simulink model "BG"  (R2014a)
settings: Solver=ode3  StartTime=0.0  StopTime=1  FixedStep=dt  MaxStep=dt  RelTol=1e-3
values from neighbouring files (symbols this model uses):
  a1 = .4    (= 0.4)    [parameters.m]
  a2 = .35    (= 0.35)    [parameters.m]
  a3 = .25    (= 0.25)    [parameters.m]
  aTc = 0.05    [parameters.m]
  dt = 1e-3    (= 0.001)    [parameters.m]
  g = 1    [parameters.m]
  K = 1    [parameters.m]
  mTc = 0.01    [parameters.m]
  OP1_0 = [ax1_0 ay1_0 0]    [parameters.m]
  OP2_0 = OP1_0 + P1P2_0    [parameters.m]
  OP3_0 = OP2_0 + P2P3_0    [parameters.m]
  OT = [xf yf 0]    [animation.m]    (also in parameters.m = [0.5 0.5 0])
  OT_cercle = [0.6 0.55 0]    [parameters.m]
  p1 = w2 + w3    (= 3)    [parameters.m]
  P1P2_0 = [ax2_0 ay2_0 0]    [parameters.m]
  p2 = w1 + w3    (= 4)    [parameters.m]
  P2P3_0 = [ax3_0 ay3_0 0]    [parameters.m]
  p3 = w2 + w1    (= 5)    [parameters.m]
  tau = 0.001    [parameters.m]
  theta1_0 = zero_vector    [parameters.m]
  theta2_0 = zero_vector    [parameters.m]
  theta3_0 = zero_vector    [parameters.m]
  Vmax = 30    [parameters.m]
  w1 = 3    [parameters.m]
  w2 = 2    [parameters.m]
  w3 = 1    [parameters.m]
  zero_vector = [0 0 0]    [parameters.m]
libraries: vrlib x9, simulink x1
(part 1 of 4)
settings Model: Creator=Armin  LastModifiedBy=Armin

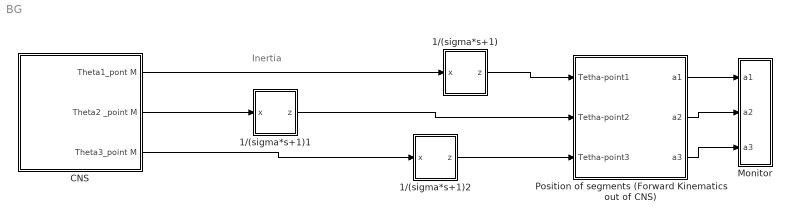
== system BG ==
  note: Inertia
  1/(sigma*s+1) : Subsystem  TreatAsAtomicUnit=on
  1/(sigma*s+1)1 : Subsystem  TreatAsAtomicUnit=on
  1/(sigma*s+1)2 : Subsystem  TreatAsAtomicUnit=on
  CNS : Subsystem
  Monitor : Subsystem
  Position of segments (Forward Kinematics out of CNS) : Subsystem
  wires:
  Position of segments (Forward Kinematics out of CNS)/1(a1) -> Monitor/1(a1)
  Position of segments (Forward Kinematics out of CNS)/2(a2) -> Monitor/2(a2)
  Position of segments (Forward Kinematics out of CNS)/3(a3) -> Monitor/3(a3)
  CNS/1(Theta1_pont M) -> 1/(sigma*s+1)/1(x)
  CNS/2(Theta2 _point M) -> 1/(sigma*s+1)1/1(x)
  CNS/3("Theta3_point M ") -> 1/(sigma*s+1)2/1(x)
  1/(sigma*s+1)/1(z) -> Position of segments (Forward Kinematics out of CNS)/1(Tetha-point1)
  1/(sigma*s+1)2/1(z) -> Position of segments (Forward Kinematics out of CNS)/3(Tetha-point3)
  1/(sigma*s+1)1/1(z) -> Position of segments (Forward Kinematics out of CNS)/2(Tetha-point2)

== system BG/1//(sigma*s+1) ==
  x : Inport
  Add : Sum  Inputs=+-
  Add1 : Sum
  Delay : Delay  DelayLength=1  InitialCondition=zero_vector
  Gain : Gain  Gain=dt
  Gain1 : Gain  Gain=0.9999999
  Gain2 : Gain  Gain=1/0.01
  z : Outport
  wires:
  Add/1 -> Gain/1
  Gain1/1 -> Add1/2, Add/2
  Delay/1 -> Gain1/1
  Gain/1 -> Gain2/1
  x/1 -> Add/1
  Add1/1 -> z/1, Delay/1
  Gain2/1 -> Add1/1

== system BG/1//(sigma*s+1)1 ==
  x : Inport
  Add : Sum  Inputs=+-
  Add1 : Sum
  Delay : Delay  DelayLength=1  InitialCondition=zero_vector
  Gain : Gain  Gain=dt
  Gain1 : Gain  Gain=0.9999999
  Gain2 : Gain  Gain=1/0.01
  z : Outport
  wires:
  Add/1 -> Gain/1
  Gain1/1 -> Add1/2, Add/2
  Delay/1 -> Gain1/1
  Gain/1 -> Gain2/1
  x/1 -> Add/1
  Add1/1 -> z/1, Delay/1
  Gain2/1 -> Add1/1

== system BG/1//(sigma*s+1)2 ==
  x : Inport
  Add : Sum  Inputs=+-
  Add1 : Sum
  Delay : Delay  DelayLength=1  InitialCondition=zero_vector
  Gain : Gain  Gain=dt
  Gain1 : Gain  Gain=0.9999999
  Gain2 : Gain  Gain=1/0.01
  z : Outport
  wires:
  Add/1 -> Gain/1
  Gain1/1 -> Add1/2, Add/2
  Delay/1 -> Gain1/1
  Gain/1 -> Gain2/1
  x/1 -> Add/1
  Add1/1 -> z/1, Delay/1
  Gain2/1 -> Add1/1

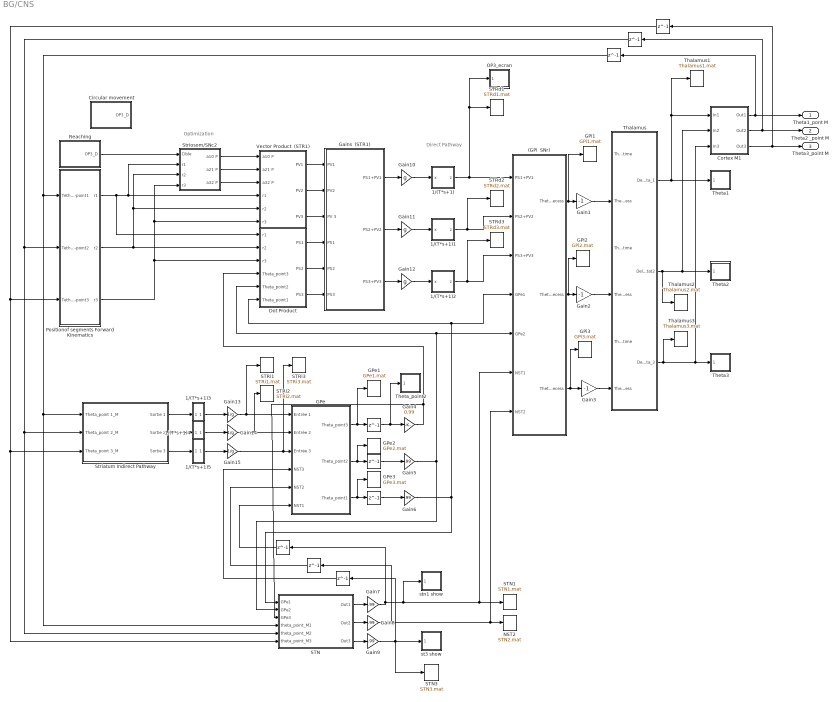
== system BG/CNS ==
  note: Direct Pathway
  note: Optimization
  " (GPi  SNr)" : Subsystem
  " Striosom/SNc2" : Subsystem
  "                                               \t\t\t\t\t\t\t" : Delay  DelayLength=1  InitialCondition=zero_vector
  "                                                                                                                                           " : Delay  DelayLength=1  InitialCondition=zero_vector
  "                                                                                                                                              \t                                                              " : Delay  DelayLength=1  InitialCondition=zero_vector
  "                                                                                                                                              \t                                                               " : Delay  DelayLength=1  InitialCondition=zero_vector
  "                                                                                                                                              \t                                                                " : Delay  DelayLength=1  InitialCondition=zero_vector
  "                                                                                                                                              \t                                                                                " : Delay  DelayLength=1  InitialCondition=zero_vector
  "                                                                                                                                              \t                                                                                    " : Delay  DelayLength=1  InitialCondition=zero_vector
  "                                                                                                                                              \t                                                                                           " : Delay  DelayLength=1  InitialCondition=zero_vector
  "                                                                                                                                                    " : Delay  DelayLength=1  InitialCondition=zero_vector
  1/(T*s+1) : Subsystem  TreatAsAtomicUnit=on
  1/(T*s+1)1 : Subsystem  TreatAsAtomicUnit=on
  1/(T*s+1)2 : Subsystem  TreatAsAtomicUnit=on
  1/(T*s+1)3 : Subsystem  TreatAsAtomicUnit=on
  1/(T*s+1)4 : Subsystem  TreatAsAtomicUnit=on
  1/(T*s+1)5 : Subsystem  TreatAsAtomicUnit=on
  Circular movement : Subsystem
  Cortex M1 : Subsystem
  Dot Product : Subsystem
  GPe : Subsystem  TreatAsAtomicUnit=on
  GPe1 : ToFile  Filename=GPe1.mat  MatrixName=gpe1
  GPe2 : ToFile  Filename=GPe2.mat  MatrixName=gpe2
  GPe3 : ToFile  Filename=GPe3.mat  MatrixName=gpe3
  GPi1 : ToFile  Filename=GPi1.mat  MatrixName=gpi1
  GPi2 : ToFile  Filename=GPi2.mat  MatrixName=gpi2
  GPi3 : ToFile  Filename=GPi3.mat  MatrixName=gpi3
  Gain1 : Gain  Gain=-1
  Gain10 : Gain  Gain=g
  Gain11 : Gain  Gain=g
  Gain12 : Gain  Gain=g
  Gain13 : Gain  Gain=1/g
  Gain14 : Gain  Gain=1/g
  Gain15 : Gain  Gain=1/g
  Gain2 : Gain  Gain=-1
  Gain3 : Gain  Gain=-1
  Gain4 : Gain  Gain=0.99
  Gain{5..9} (5 alike) : Gain  Gain=.99
  Gains  (STR1) : Subsystem
  NST2 : ToFile  Filename=STN2.mat  MatrixName=stn2
  OP3_ecran : Subsystem
  Positionof segments Forward Kinematics : Subsystem
  Reaching : Subsystem
  STN : Subsystem
  STN1 : ToFile  Filename=STN1.mat  MatrixName=stn1
  STN3 : ToFile  Filename=STN3.mat  MatrixName=stn3
  STRd1 : ToFile  Filename=STRd1.mat  MatrixName=strd1
  STRd2 : ToFile  Filename=STRd2.mat  MatrixName=strd2
  STRd3 : ToFile  Filename=STRd3.mat  MatrixName=strd3
  STRi1 : ToFile  Filename=STRi1.mat  MatrixName=stri1
  STRi2 : ToFile  Filename=STRi2.mat  MatrixName=stri2
  STRi3 : ToFile  Filename=STRi3.mat  MatrixName=stri3
  Striatum Indirect Pathway : Subsystem  TreatAsAtomicUnit=on
  Thalamus : Subsystem
  Thalamus1 : ToFile  Filename=Thalamus1.mat  MatrixName=thalamus1
  Thalamus2 : ToFile  Filename=Thalamus2.mat  MatrixName=thalamus2
  Thalamus3 : ToFile  Filename=Thalamus3.mat  MatrixName=thalamus3
  Theta1 : Subsystem
  Theta2 : Subsystem
  Theta3 : Subsystem
  Theta_point2 : Subsystem
  Vector Product  (STR1) : Subsystem
  st3 show : Subsystem
  stn1 show : Subsystem
  Theta1_pont M : Outport
  Theta2 _point M : Outport  Port=2
  "Theta3_point M " : Outport  Port=3
  wires:
  Thalamus/1(Delta-theta_1) -> Thalamus1/1, Cortex M1/1(In1), Theta1/1(In_vec)
  Thalamus/2(Delta_thetat2) -> Thalamus2/1, Theta2/1(In_vec), Cortex M1/2(In2)
  Thalamus/3(Delta_theta_3) -> Thalamus3/1, Theta3/1(In_vec), Cortex M1/3(In3)
  Vector Product  (STR1)/2(PV2) -> Gains  (STR1)/2(PV2)
  Vector Product  (STR1)/3(PV3) -> Gains  (STR1)/3(PV 3)
  Vector Product  (STR1)/1(PV1) -> Gains  (STR1)/1(PV1)
  " Striosom/SNc2"/1(a10 P) -> Vector Product  (STR1)/1(a10 P)
  " Striosom/SNc2"/2(a21 P) -> Vector Product  (STR1)/2(a21 P)
  " Striosom/SNc2"/3(a32 P) -> Vector Product  (STR1)/3(a32 P)
  Dot Product/2(PS2) -> Gains  (STR1)/5(PS2)
  Dot Product/3(PS3) -> Gains  (STR1)/6(PS3)
  Dot Product/1(PS1) -> Gains  (STR1)/4(PS1)
  " (GPi  SNr)"/1(Theta1_Necess) -> GPi1/1, Gain1/1
  " (GPi  SNr)"/2(Theta2_Necess) -> GPi2/1, Gain2/1
  " (GPi  SNr)"/3(Theta3_Necess) -> GPi3/1, Gain3/1
  Cortex M1/2(Out2) -> Theta2 _point M/1, "                                                                                                                                           "/1
  Cortex M1/1(Out1) -> "                                                                                                                                                    "/1, Theta1_pont M/1
  Cortex M1/3(Out3) -> "Theta3_point M "/1, "                                               \t\t\t\t\t\t\t"/1
  Gain3/1 -> Thalamus/6(Theta3_necess)
  Gain2/1 -> Thalamus/4(Theta2_necess)
  Gain1/1 -> Thalamus/2(Theta1_necess)
  GPe/3(Theta_point1) -> GPe3/1, "                                                                                                                                              \t                                                              "/1
  GPe/2(Theta_point2) -> GPe2/1, "                                                                                                                                              \t                                                                "/1
  GPe/1(Theta_point3) -> GPe1/1, "                                                                                                                                              \t                                                               "/1
  "                                                                                                                                              \t                                                              "/1 -> Gain6/1
  "                                                                                                                                              \t                                                                "/1 -> Gain5/1
  "                                                                                                                                              \t                                                                                    "/1 -> GPe/6(NST1)
  "                                                                                                                                              \t                                                                                "/1 -> GPe/5("NST2 ")
  STN/3(Out3) -> Gain9/1
  STN/1(Out1) -> Gain7/1
  STN/2(Out2) -> Gain8/1
  "                                                                                                                                              \t                                                               "/1 -> Theta_point2/1(In_vec), Gain4/1
  "                                                                                                                                              \t                                                                                           "/1 -> GPe/4(NST3)
  Striatum Indirect Pathway/1(Sortie 1) -> 1/(T*s+1)3/1(x)
  Positionof segments Forward Kinematics/1(r1) -> " Striosom/SNc2"/2(r1), Vector Product  (STR1)/4(r1), Dot Product/1(r1)
  Positionof segments Forward Kinematics/2(r2) -> " Striosom/SNc2"/3(r2), Vector Product  (STR1)/5(r2), Dot Product/2(r2)
  Positionof segments Forward Kinematics/3(r3) -> " Striosom/SNc2"/4(r3), Vector Product  (STR1)/6(r3), Dot Product/3(r3)
  Gains  (STR1)/1(PS1+PV1) -> Gain10/1
  Gains  (STR1)/2(PS2+PV2) -> Gain11/1
  Gains  (STR1)/3(PS3+PV3) -> Gain12/1
  Gain6/1 -> " (GPi  SNr)"/4(GPe1), Dot Product/6(Theta_point1), STN/1(GPe1)
  Gain5/1 -> " (GPi  SNr)"/5(GPe2), Dot Product/5(Theta_point2), STN/2(GPe2)
  Gain7/1 -> stn1 show/1(In_vec), " (GPi  SNr)"/6(NST1), STN1/1, "                                                                                                                                              \t                                                                                    "/1
  Gain8/1 -> "                                                                                                                                              \t                                                                                "/1, " (GPi  SNr)"/7(NST2), NST2/1
  "                                                                                                                                                    "/1 -> STN/4(theta_point_M1), Striatum Indirect Pathway/1(Theta_point 1_M), Positionof segments Forward Kinematics/1(Tetha-point1)
  "                                                                                                                                           "/1 -> STN/5(theta_point_M2), Striatum Indirect Pathway/2(Theta_point 2_M), Positionof segments Forward Kinematics/2(Tetha-point2)
  "                                               \t\t\t\t\t\t\t"/1 -> STN/6(theta_point_M3), Striatum Indirect Pathway/3(Theta_point 3_M), Positionof segments Forward Kinematics/3(Tetha-point3)
  Striatum Indirect Pathway/2(Sortie 2) -> 1/(T*s+1)4/1(x)
  Striatum Indirect Pathway/3(Sortie 3) -> 1/(T*s+1)5/1(x)
  Gain4/1 -> STN/3(GPe3), Dot Product/4(Theta_point3)
  Gain9/1 -> "                                                                                                                                              \t                                                                                           "/1, st3 show/1(In_vec), STN3/1
  Gain10/1 -> 1/(T*s+1)/1(x)
  Gain11/1 -> 1/(T*s+1)1/1(x)
  Gain12/1 -> 1/(T*s+1)2/1(x)
  Gain14/1 -> GPe/2(Entrée 2), STRi2/1
  Gain15/1 -> STRi3/1, GPe/3(Entrée 3)
  1/(T*s+1)/1(z) -> OP3_ecran/1(In_vec), STRd1/1, " (GPi  SNr)"/1(PS1+PV1)
  1/(T*s+1)1/1(z) -> STRd2/1, " (GPi  SNr)"/2(PS2+PV2)
  1/(T*s+1)2/1(z) -> STRd3/1, " (GPi  SNr)"/3(PS3+PV3)
  Gain13/1 -> STRi1/1, GPe/1(Entrée 1)
  Reaching/1(OP3_D) -> " Striosom/SNc2"/1(Cible)
  1/(T*s+1)3/1(z) -> Gain13/1
  1/(T*s+1)4/1(z) -> Gain14/1
  1/(T*s+1)5/1(z) -> Gain15/1

== system BG/Monitor ==
  a1 : Inport
  a2 : Inport  Port=2
  a3 : Inport  Port=3
  "                       " : Sum
  "                        " : Sum
  OP1 : ToFile  Filename=P1.mat  MatrixName=P1
  OP1_ecran : Subsystem
  OP2 : ToFile  Filename=P2.mat  MatrixName=P2
  OP2_ecran : Subsystem
  OP3 : ToFile  Filename=P3.mat  MatrixName=P3
  OP3_ecran : Subsystem
  wires:
  a1/1 -> "                       "/1, OP1_ecran/1(In_vec), OP1/1
  a2/1 -> "                       "/2
  "                       "/1 -> OP2/1, "                        "/1, OP2_ecran/1(In_vec)
  a3/1 -> "                        "/2
  "                        "/1 -> OP3_ecran/1(In_vec), OP3/1

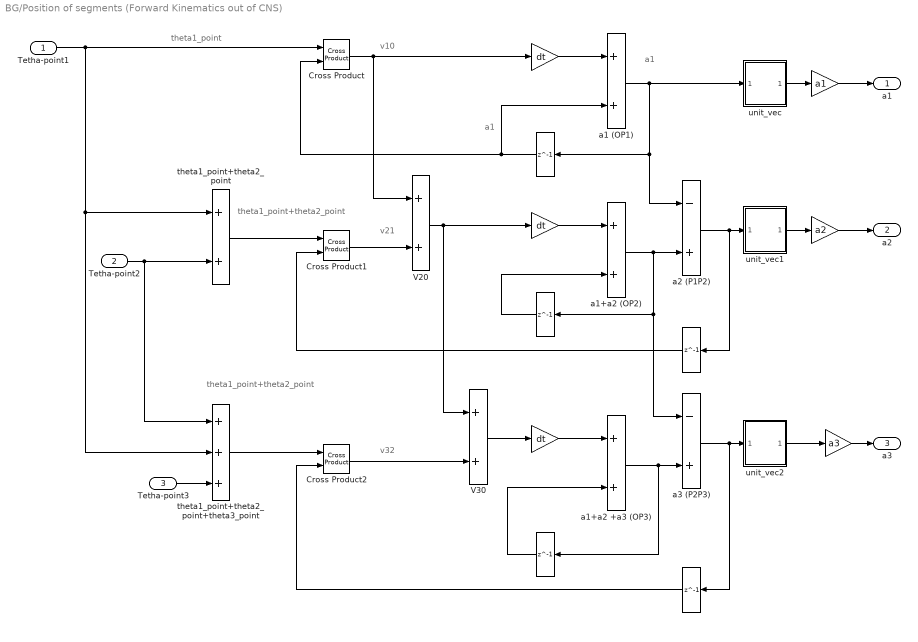
== system BG/Position of segments (Forward Kinematics out of CNS) ==
  note: theta1_point
  note: a1
  note: v10
  note: a1
  note: theta1_point+theta2_point
  note: v21
  note: theta1_point+theta2_point
  note: v32
  Tetha-point1 : Inport
  Tetha-point2 : Inport  Port=2
  Tetha-point3 : Inport  Port=3
  " " : Delay  DelayLength=1  InitialCondition=OP1_0
  "  " : Delay  DelayLength=1  InitialCondition=OP2_0
  "        " : Gain  Gain=dt
  "         " : Gain  Gain=a1
  "          " : Delay  DelayLength=1  InitialCondition=OP3_0
  "              " : Gain  Gain=a2
  "                  " : Delay  DelayLength=1  InitialCondition=P1P2_0
  "                         " : Gain  Gain=a3
  "                                  " : Gain  Gain=dt
  "                                                             " : Gain  Gain=dt
  "                                                              " : Delay  DelayLength=1  InitialCondition=P2P3_0
  "Cross Product " : vrlib/Utilities/Cross Product
  Cross Product1 : vrlib/Utilities/Cross Product
  Cross Product2 : vrlib/Utilities/Cross Product
  V20 : Sum
  V30 : Sum
  a1 (OP1) : Sum
  a1+a2 (OP2) : Sum
  a1+a2 +a3 (OP3) : Sum
  a2 (P1P2) : Sum  Inputs=-+
  a3 (P2P3) : Sum  Inputs=-+
  theta1_point+theta2_point : Sum
  theta1_point+theta2_point+theta3_point : Sum  Inputs=+++
  unit_vec : Subsystem
  unit_vec1 : Subsystem
  unit_vec2 : Subsystem
  a1 : Outport
  a2 : Outport  Port=2
  a3 : Outport  Port=3
  wires:
  "        "/1 -> a1 (OP1)/1
  " "/1 -> "Cross Product "/2, a1 (OP1)/2
  Tetha-point1/1 -> "Cross Product "/1, theta1_point+theta2_point/1, theta1_point+theta2_point+theta3_point/2
  Tetha-point2/1 -> theta1_point+theta2_point+theta3_point/1, theta1_point+theta2_point/2
  theta1_point+theta2_point/1 -> Cross Product1/1
  Tetha-point3/1 -> theta1_point+theta2_point+theta3_point/3
  theta1_point+theta2_point+theta3_point/1 -> Cross Product2/1
  V20/1 -> "                                  "/1, V30/1
  "                                  "/1 -> a1+a2 (OP2)/1
  a1+a2 (OP2)/1 -> a2 (P1P2)/2, a3 (P2P3)/1, "  "/1
  "  "/1 -> a1+a2 (OP2)/2
  "                  "/1 -> Cross Product1/2
  V30/1 -> "                                                             "/1
  a1+a2 +a3 (OP3)/1 -> a3 (P2P3)/2, "          "/1
  "          "/1 -> a1+a2 +a3 (OP3)/2
  "                                                              "/1 -> Cross Product2/2
  "                                                             "/1 -> a1+a2 +a3 (OP3)/1
  "Cross Product "/1 -> V20/1, "        "/1
  Cross Product1/1 -> V20/2
  Cross Product2/1 -> V30/2
  a1 (OP1)/1 -> a2 (P1P2)/1, " "/1, unit_vec/1(vec1)
  a2 (P1P2)/1 -> "                  "/1, unit_vec1/1(vec1)
  a3 (P2P3)/1 -> unit_vec2/1(vec1), "                                                              "/1
  unit_vec/1(vec2) -> "         "/1
  "         "/1 -> a1/1
  unit_vec1/1(vec2) -> "              "/1
  "              "/1 -> a2/1
  "                         "/1 -> a3/1
  unit_vec2/1(vec2) -> "                         "/1

== system BG/CNS/ (GPi  SNr) ==
  PS1+PV1 : Inport
  PS2+PV2 : Inport  Port=2
  PS3+PV3 : Inport  Port=3
  GPe1 : Inport  Port=4
  GPe2 : Inport  Port=5
  NST1 : Inport  Port=6
  NST2 : Inport  Port=7
  "                                  " : Sum  Inputs=--+
  "                                       " : Sum  Inputs=--+
  Gain : Gain  Gain=-1
  Integrateur : Subsystem
  Integrateur1 : Subsystem
  Integrateur2 : Subsystem
  theta_point1 : ToFile  Filename=theta_point1.mat  MatrixName=theta_point1
  theta_point2 : ToFile  Filename=theta_point2.mat  MatrixName=theta_point2
  theta_point3 : ToFile  Filename=theta_point3.mat  MatrixName=theta_point3
  Theta1_Necess : Outport
  Theta2_Necess : Outport  Port=2
  Theta3_Necess : Outport  Port=3
  wires:
  PS1+PV1/1 -> Gain/1
  "                                       "/1 -> theta_point2/1, Integrateur1/1(In1)
  PS2+PV2/1 -> "                                       "/1
  PS3+PV3/1 -> "                                  "/1
  "                                  "/1 -> theta_point3/1, Integrateur2/1(In1)
  GPe1/1 -> "                                       "/2
  GPe2/1 -> "                                  "/2
  Integrateur1/1(Out1) -> Theta2_Necess/1
  Integrateur2/1(Out1) -> Theta3_Necess/1
  NST1/1 -> "                                       "/3
  NST2/1 -> "                                  "/3
  Gain/1 -> theta_point1/1, Integrateur/1(In1)
  Integrateur/1(Out1) -> Theta1_Necess/1

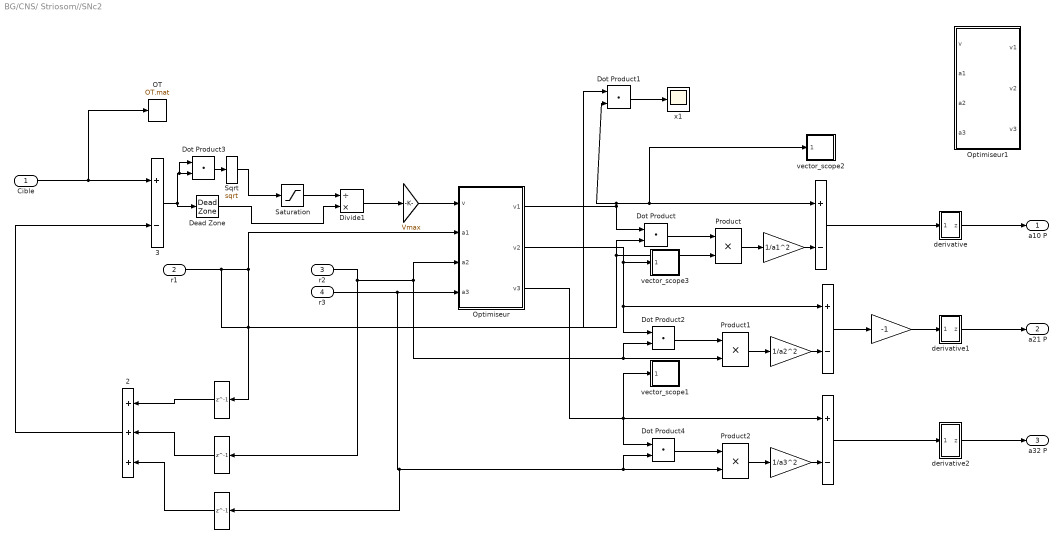
== system BG/CNS/ Striosom//SNc2 ==
  Cible : Inport
  r1 : Inport  Port=2
  r2 : Inport  Port=3
  r3 : Inport  Port=4
  "                           " : Delay  DelayLength=1  InitialCondition=OP1_0
  "                            " : Delay  DelayLength=1  InitialCondition=P1P2_0
  "                             " : Delay  DelayLength=1  InitialCondition=P2P3_0
  "                                                                                                   " : Gain  Gain=1/a1^2
  "                                                                                                    " : Sum  Inputs=+-
  "                                                                                                      " : Gain  Gain=1/a2^2
  "                                                                                                       " : Gain  Gain=-1
  "                                                                                                                                     " : Sum  Inputs=+-
  "                                                                                                                                                " : Gain  Gain=Vmax
  "                                                                                                                                                           " : Gain  Gain=1/a3^2
  "                                                                                                                                                                                      " : Sum  Inputs=+-
  "                                                                                                    2" : Sum  Inputs=+++
  "                                                                                                    3" : Sum  Inputs=+-
  Dead Zone : DeadZone  LowerValue=-0.001  UpperValue=0.001  SaturateOnIntegerOverflow=on
  Divide1 : Product  Inputs=/*
  Dot Product{,1..4} (5 alike) : DotProduct  InputSameDT=on  OutDataTypeStr=Inherit: Inherit via internal rule
  OT : ToFile  Filename=OT.mat  MatrixName=T
  Optimiseur : Subsystem
  Optimiseur1 : Subsystem
  Product : Product
  Product1 : Product
  Product2 : Product
  Saturation : Saturate  UpperLimit=2  LowerLimit=0.1
  Sqrt : Sqrt  SaturateOnIntegerOverflow=on
  derivative : Subsystem  TreatAsAtomicUnit=on
  derivative1 : Subsystem  TreatAsAtomicUnit=on
  derivative2 : Subsystem  TreatAsAtomicUnit=on
  vector_scope1 : Subsystem
  vector_scope2 : Subsystem
  vector_scope3 : Subsystem
  x1 : Scope
      settings: SaveName=ScopeData6
  a10 P : Outport
  a21 P : Outport  Port=2
  a32 P : Outport  Port=3
  wires:
  derivative/1(z) -> a10 P/1
  derivative1/1(z) -> a21 P/1
  derivative2/1(z) -> a32 P/1
  Optimiseur/1(v1) -> "                                                                                                    "/1, vector_scope2/1(In_vec), Dot Product1/2, Dot Product/1
  Dot Product/1 -> Product/1
  Product/1 -> "                                                                                                   "/1
  "                                                                                                   "/1 -> "                                                                                                    "/2
  "                                                                                                    "/1 -> derivative/1(x)
  Optimiseur/2(v2) -> Dot Product2/1, "                                                                                                                                     "/1, vector_scope3/1(In_vec)
  Dot Product2/1 -> Product1/1
  Product1/1 -> "                                                                                                      "/1
  "                                                                                                      "/1 -> "                                                                                                                                     "/2
  r2/1 -> "                            "/1, Optimiseur/3(a2), Dot Product2/2, Product1/2
  "                                                                                                                                     "/1 -> "                                                                                                       "/1
  Optimiseur/3(v3) -> vector_scope1/1(In_vec), Dot Product4/1, "                                                                                                                                                                                      "/1
  Dot Product4/1 -> Product2/1
  Product2/1 -> "                                                                                                                                                           "/1
  "                                                                                                                                                           "/1 -> "                                                                                                                                                                                      "/2
  r3/1 -> Optimiseur/4(a3), "                             "/1, Dot Product4/2, Product2/2
  "                                                                                                                                                                                      "/1 -> derivative2/1(x)
  r1/1 -> Dot Product1/1, Optimiseur/2(a1), "                           "/1, Product/2, Dot Product/2
  Dot Product1/1 -> x1/1
  "                                                                                                       "/1 -> derivative1/1(x)
  "                                                                                                                                                "/1 -> Optimiseur/1(v)
  "                           "/1 -> "                                                                                                    2"/1
  "                            "/1 -> "                                                                                                    2"/2
  "                             "/1 -> "                                                                                                    2"/3
  "                                                                                                    2"/1 -> "                                                                                                    3"/2
  Divide1/1 -> "                                                                                                                                                "/1
  Dot Product3/1 -> Sqrt/1
  "                                                                                                    3"/1 -> Dot Product3/1, Dot Product3/2, Dead Zone/1
  Sqrt/1 -> Saturation/1
  Saturation/1 -> Divide1/1
  Dead Zone/1 -> Divide1/2
  Cible/1 -> OT/1, "                                                                                                    3"/1

== system BG/CNS/1//(T*s+1) ==
  x : Inport
  Add : Sum  Inputs=+-
  Add1 : Sum
  Delay : Delay  DelayLength=1  InitialCondition=OP3_0
  Gain : Gain  Gain=dt
  Gain2 : Gain  Gain=1/tau
  z : Outport
  wires:
  Add/1 -> Gain/1
  Delay/1 -> Add1/2, Add/2
  Gain/1 -> Gain2/1
  x/1 -> Add/1
  Add1/1 -> z/1, Delay/1
  Gain2/1 -> Add1/1

== system BG/CNS/1//(T*s+1)1 ==
  x : Inport
  Add : Sum  Inputs=+-
  Add1 : Sum
  Delay : Delay  DelayLength=1  InitialCondition=OP3_0
  Gain : Gain  Gain=dt
  Gain2 : Gain  Gain=1/tau
  z : Outport
  wires:
  Add/1 -> Gain/1
  Delay/1 -> Add1/2, Add/2
  Gain/1 -> Gain2/1
  x/1 -> Add/1
  Add1/1 -> z/1, Delay/1
  Gain2/1 -> Add1/1

== system BG/CNS/1//(T*s+1)2 ==
  x : Inport
  Add : Sum  Inputs=+-
  Add1 : Sum
  Delay : Delay  DelayLength=1  InitialCondition=OP3_0
  Gain : Gain  Gain=dt
  Gain2 : Gain  Gain=1/tau
  z : Outport
  wires:
  Add/1 -> Gain/1
  Delay/1 -> Add1/2, Add/2
  Gain/1 -> Gain2/1
  x/1 -> Add/1
  Add1/1 -> z/1, Delay/1
  Gain2/1 -> Add1/1

== system BG/CNS/1//(T*s+1)3 ==
  x : Inport
  Add : Sum  Inputs=+-
  Add1 : Sum
  Delay : Delay  DelayLength=1  InitialCondition=OP3_0
  Gain : Gain  Gain=dt
  Gain2 : Gain  Gain=1/tau
  z : Outport
  wires:
  Add/1 -> Gain/1
  Delay/1 -> Add1/2, Add/2
  Gain/1 -> Gain2/1
  x/1 -> Add/1
  Add1/1 -> z/1, Delay/1
  Gain2/1 -> Add1/1

== system BG/CNS/1//(T*s+1)4 ==
  x : Inport
  Add : Sum  Inputs=+-
  Add1 : Sum
  Delay : Delay  DelayLength=1  InitialCondition=OP3_0
  Gain : Gain  Gain=dt
  Gain2 : Gain  Gain=1/tau
  z : Outport
  wires:
  Add/1 -> Gain/1
  Delay/1 -> Add1/2, Add/2
  Gain/1 -> Gain2/1
  x/1 -> Add/1
  Add1/1 -> z/1, Delay/1
  Gain2/1 -> Add1/1

== system BG/CNS/1//(T*s+1)5 ==
  x : Inport
  Add : Sum  Inputs=+-
  Add1 : Sum
  Delay : Delay  DelayLength=1  InitialCondition=OP3_0
  Gain : Gain  Gain=dt
  Gain2 : Gain  Gain=1/tau
  z : Outport
  wires:
  Add/1 -> Gain/1
  Delay/1 -> Add1/2, Add/2
  Gain/1 -> Gain2/1
  x/1 -> Add/1
  Add1/1 -> z/1, Delay/1
  Gain2/1 -> Add1/1

== system BG/CNS/Circular movement ==
  1/(T*s+1) : Subsystem  TreatAsAtomicUnit=on
  1/(T*s+1)1 : Subsystem  TreatAsAtomicUnit=on
  1/(T*s+1)2 : Subsystem  TreatAsAtomicUnit=on
  Add1 : Sum  Inputs=++-
  Theta_point1 : Subsystem
  Theta_point2 : Subsystem
  Theta_point3 : Subsystem
  la premiere cible : Step  Time=0  Before=OP3_0  After=OT_cercle  SampleTime=0
  la premiere cible1 : Step  Time=0.06  Before=zero_vector  After=OT_cercle  SampleTime=0
  le cercle : FromFile  FileName=circle_motion.mat  SampleTime=0
  OP3_D : Outport
  wires:
  le cercle/1 -> Add1/1, Theta_point1/1(In_vec)
  la premiere cible/1 -> 1/(T*s+1)/1(x)
  1/(T*s+1)/1(z) -> Add1/2
  la premiere cible1/1 -> 1/(T*s+1)1/1(x)
  1/(T*s+1)1/1(z) -> Add1/3, Theta_point3/1(In_vec)
  Add1/1 -> 1/(T*s+1)2/1(x)
  1/(T*s+1)2/1(z) -> Theta_point2/1(In_vec), OP3_D/1

== system BG/CNS/Cortex M1 ==
  In1 : Inport
  In2 : Inport  Port=2
  In3 : Inport  Port=3
  derivative : Subsystem  TreatAsAtomicUnit=on
  derivative1 : Subsystem  TreatAsAtomicUnit=on
  derivative2 : Subsystem  TreatAsAtomicUnit=on
  Out1 : Outport
  Out2 : Outport  Port=2
  Out3 : Outport  Port=3
  wires:
  In1/1 -> derivative/1(x)
  derivative/1(z) -> Out1/1
  In2/1 -> derivative1/1(x)
  derivative1/1(z) -> Out2/1
  In3/1 -> derivative2/1(x)
  derivative2/1(z) -> Out3/1

== system BG/CNS/Dot Product ==
  r1 : Inport
  r2 : Inport  Port=2
  r3 : Inport  Port=3
  Theta_point3 : Inport  Port=4
  Theta_point2 : Inport  Port=5
  Theta_point1 : Inport  Port=6
  "                                                      " : Sum  Inputs=---
  "                                                                     " : Sum  Inputs=--
  Dot Product : DotProduct  InputSameDT=on  OutDataTypeStr=Inherit: Inherit via internal rule
  Dot Product1 : DotProduct  InputSameDT=on  OutDataTypeStr=Inherit: Inherit via internal rule
  Dot Product2 : DotProduct  InputSameDT=on  OutDataTypeStr=Inherit: Inherit via internal rule
  Gain13 : Gain  Gain=-1
  Product : Product
  Product1 : Product
  Product2 : Product
  PS1 : Outport
  PS2 : Outport  Port=2
  PS3 : Outport  Port=3
  wires:
  Dot Product/1 -> Product/1
  Product/1 -> PS2/1
  r3/1 -> Dot Product1/2, Product1/2
  Dot Product1/1 -> Product1/1
  Product1/1 -> PS3/1
  "                                                      "/1 -> Dot Product1/1
  Theta_point2/1 -> "                                                                     "/2, "                                                      "/2
  r2/1 -> Dot Product/2, Product/2
  Theta_point3/1 -> "                                                      "/3
  "                                                                     "/1 -> Dot Product/1
  Dot Product2/1 -> Product2/1
  Product2/1 -> PS1/1
  r1/1 -> Dot Product2/2, Product2/2
  Theta_point1/1 -> Gain13/1, "                                                                     "/1, "                                                      "/1
  Gain13/1 -> Dot Product2/1

== system BG/CNS/GPe ==
  Entrée 1 : Inport
  Entrée 2 : Inport  Port=2
  Entrée 3 : Inport  Port=3
  NST3 : Inport  Port=4
  "NST2 " : Inport  Port=5
  NST1 : Inport  Port=6
  "                                                    " : Sum  Inputs=-+
  "                                                       " : Sum  Inputs=-+
  "                                                        " : Sum  Inputs=-+
  1/(sigma*s+1) : Subsystem  TreatAsAtomicUnit=on
  1/(sigma*s+1)1 : Subsystem  TreatAsAtomicUnit=on
  1/(sigma*s+1)2 : Subsystem  TreatAsAtomicUnit=on
  Gain1 : Gain
  Gain11 : Gain
  Gain2 : Gain
  Theta_point4 : Subsystem
  Theta_point3 : Outport
  Theta_point2 : Outport  Port=2
  Theta_point1 : Outport  Port=3
  wires:
  "                                                    "/1 -> Theta_point4/1(In_vec), 1/(sigma*s+1)/1(x)
  Entrée 1/1 -> "                                                    "/1
  Entrée 2/1 -> "                                                       "/1
  Entrée 3/1 -> "                                                        "/1
  "                                                        "/1 -> 1/(sigma*s+1)2/1(x)
  "                                                       "/1 -> 1/(sigma*s+1)1/1(x)
  NST3/1 -> "                                                        "/2
  "NST2 "/1 -> "                                                       "/2
  NST1/1 -> "                                                    "/2
  1/(sigma*s+1)/1(z) -> Gain11/1
  1/(sigma*s+1)1/1(z) -> Gain1/1
  1/(sigma*s+1)2/1(z) -> Gain2/1
  Gain11/1 -> Theta_point1/1
  Gain1/1 -> Theta_point2/1
  Gain2/1 -> Theta_point3/1

== system BG/CNS/Gains  (STR1) ==
  PV1 : Inport
  PV2 : Inport  Port=2
  PV 3 : Inport  Port=3
  PS1 : Inport  Port=4
  PS2 : Inport  Port=5
  PS3 : Inport  Port=6
  Normaliser : Subsystem
  PS1+PV1 : Outport
  PS2+PV2 : Outport  Port=2
  PS3+PV3 : Outport  Port=3
  wires:
  PV2/1 -> Normaliser/5(PV2)
  PS2/1 -> Normaliser/2(PS2)
  PV1/1 -> Normaliser/4(PV1)
  PS1/1 -> Normaliser/1(PS1)
  PV 3/1 -> Normaliser/6(PV 3)
  PS3/1 -> Normaliser/3(PS3)
  Normaliser/1(PS1+PV1) -> PS1+PV1/1
  Normaliser/2(PS2+PV2) -> PS2+PV2/1
  Normaliser/3(PS3+PV3) -> PS3+PV3/1

== system BG/CNS/OP3_ecran ==
  In_vec : Inport
  Demux : Demux  Outputs=3
  x : Scope
  y : Scope
      settings: SaveName=ScopeData2
  z : Scope
      settings: SaveName=ScopeData3
  wires:
  In_vec/1 -> Demux/1
  Demux/1 -> x/1
  Demux/2 -> y/1
  Demux/3 -> z/1

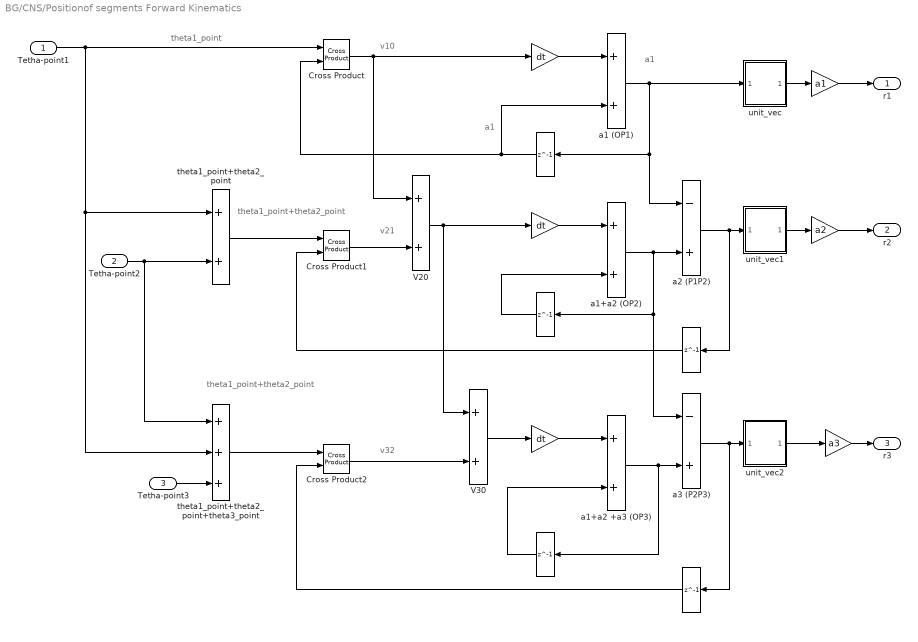
== system BG/CNS/Positionof segments Forward Kinematics ==
  note: theta1_point
  note: a1
  note: v10
  note: a1
  note: theta1_point+theta2_point
  note: v21
  note: theta1_point+theta2_point
  note: v32
  Tetha-point1 : Inport
  Tetha-point2 : Inport  Port=2
  Tetha-point3 : Inport  Port=3
  " " : Delay  DelayLength=1  InitialCondition=OP1_0
  "  " : Delay  DelayLength=1  InitialCondition=OP2_0
  "        " : Gain  Gain=dt
  "         " : Gain  Gain=a1
  "          " : Delay  DelayLength=1  InitialCondition=OP3_0
  "              " : Gain  Gain=a2
  "                  " : Delay  DelayLength=1  InitialCondition=P1P2_0
  "                         " : Gain  Gain=a3
  "                                  " : Gain  Gain=dt
  "                                                             " : Gain  Gain=dt
  "                                                              " : Delay  DelayLength=1  InitialCondition=P2P3_0
  "Cross Product " : vrlib/Utilities/Cross Product
  Cross Product1 : vrlib/Utilities/Cross Product
  Cross Product2 : vrlib/Utilities/Cross Product
  V20 : Sum
  V30 : Sum
  a1 (OP1) : Sum
  a1+a2 (OP2) : Sum
  a1+a2 +a3 (OP3) : Sum
  a2 (P1P2) : Sum  Inputs=-+
  a3 (P2P3) : Sum  Inputs=-+
  theta1_point+theta2_point : Sum
  theta1_point+theta2_point+theta3_point : Sum  Inputs=+++
  unit_vec : Subsystem
  unit_vec1 : Subsystem
  unit_vec2 : Subsystem
  r1 : Outport
  r2 : Outport  Port=2
  r3 : Outport  Port=3
  wires:
  "        "/1 -> a1 (OP1)/1
  " "/1 -> "Cross Product "/2, a1 (OP1)/2
  Tetha-point1/1 -> "Cross Product "/1, theta1_point+theta2_point/1, theta1_point+theta2_point+theta3_point/2
  Tetha-point2/1 -> theta1_point+theta2_point+theta3_point/1, theta1_point+theta2_point/2
  theta1_point+theta2_point/1 -> Cross Product1/1
  Tetha-point3/1 -> theta1_point+theta2_point+theta3_point/3
  theta1_point+theta2_point+theta3_point/1 -> Cross Product2/1
  V20/1 -> "                                  "/1, V30/1
  "                                  "/1 -> a1+a2 (OP2)/1
  a1+a2 (OP2)/1 -> a2 (P1P2)/2, a3 (P2P3)/1, "  "/1
  "  "/1 -> a1+a2 (OP2)/2
  "                  "/1 -> Cross Product1/2
  V30/1 -> "                                                             "/1
  a1+a2 +a3 (OP3)/1 -> a3 (P2P3)/2, "          "/1
  "          "/1 -> a1+a2 +a3 (OP3)/2
  "                                                              "/1 -> Cross Product2/2
  "                                                             "/1 -> a1+a2 +a3 (OP3)/1
  "Cross Product "/1 -> V20/1, "        "/1
  Cross Product1/1 -> V20/2
  Cross Product2/1 -> V30/2
  a1 (OP1)/1 -> a2 (P1P2)/1, " "/1, unit_vec/1(vec1)
  a2 (P1P2)/1 -> "                  "/1, unit_vec1/1(vec1)
  a3 (P2P3)/1 -> unit_vec2/1(vec1), "                                                              "/1
  unit_vec/1(vec2) -> "         "/1
  "         "/1 -> r1/1
  unit_vec1/1(vec2) -> "              "/1
  "              "/1 -> r2/1
  "                         "/1 -> r3/1
  unit_vec2/1(vec2) -> "                         "/1

== system BG/CNS/Reaching ==
  1/(T*s+1) : Subsystem  TreatAsAtomicUnit=on
  Theta_point1 : Subsystem
  derivative : Subsystem  TreatAsAtomicUnit=on
  la premiere cible : Step  Time=0.1  Before=OP3_0  After=OT  SampleTime=0
  vitesse : Subsystem
  OP3_D : Outport
  wires:
  1/(T*s+1)/1(z) -> derivative/1(x), OP3_D/1
  la premiere cible/1 -> Theta_point1/1(In_vec), 1/(T*s+1)/1(x)
  derivative/1(z) -> vitesse/1(In_vec)

== system BG/CNS/STN ==
  GPe1 : Inport
  GPe2 : Inport  Port=2
  GPe3 : Inport  Port=3
  theta_point_M1 : Inport  Port=4
  theta_point_M2 : Inport  Port=5
  theta_point_M3 : Inport  Port=6
  1/(sigma*s+1) : Subsystem  TreatAsAtomicUnit=on
  1/(sigma*s+1)1 : Subsystem  TreatAsAtomicUnit=on
  1/(sigma*s+1)2 : Subsystem  TreatAsAtomicUnit=on
  Add1 : Sum  Inputs=+-
  Add2 : Sum  Inputs=+++-
  Add3 : Sum  Inputs=++-
  Add4 : Sum
  Add5 : Sum
  Add6 : Sum
  Gain : Gain  Gain=K
  Gain1 : Gain  Gain=0.1
  Gain2 : Gain  Gain=K
  Gain3 : Gain  Gain=K
  Gain4 : Gain  Gain=0.1
  Gain5 : Gain  Gain=0.1
  Gain6 : Gain
  Gain7 : Gain
  Gain8 : Gain
  s/(Ts+1) : Subsystem  TreatAsAtomicUnit=on
  s/(Ts+1)2 : Subsystem  TreatAsAtomicUnit=on
  s/(Ts+1)3 : Subsystem  TreatAsAtomicUnit=on
  Out1 : Outport
  Out2 : Outport  Port=2
  Out3 : Outport  Port=3
  wires:
  GPe2/1 -> Add3/3
  1/(sigma*s+1)2/1(z) -> Gain8/1
  GPe3/1 -> Add2/4
  Add4/1 -> 1/(sigma*s+1)/1(x)
  Add6/1 -> 1/(sigma*s+1)1/1(x)
  Add5/1 -> 1/(sigma*s+1)2/1(x)
  Gain/1 -> Add4/1
  Add1/1 -> s/(Ts+1)/1(In1), Gain/1
  theta_point_M1/1 -> Add3/1, Add2/1, Add1/1
  GPe1/1 -> Add1/2
  Gain3/1 -> Add6/1
  Add3/1 -> s/(Ts+1)3/1(In1), Gain3/1
  theta_point_M2/1 -> Add2/2, Add3/2
  Add2/1 -> s/(Ts+1)2/1(In1), Gain2/1
  Gain2/1 -> Add5/1
  theta_point_M3/1 -> Add2/3
  s/(Ts+1)2/1(Out1) -> Gain5/1
  s/(Ts+1)3/1(Out1) -> Gain4/1
  s/(Ts+1)/1(Out1) -> Gain1/1
  1/(sigma*s+1)/1(z) -> Gain6/1
  1/(sigma*s+1)1/1(z) -> Gain7/1
  Gain8/1 -> Out3/1
  Gain7/1 -> Out2/1
  Gain6/1 -> Out1/1
  Gain4/1 -> Add6/2
  Gain5/1 -> Add5/2
  Gain1/1 -> Add4/2

== system BG/CNS/Striatum Indirect Pathway ==
  Theta_point 1_M : Inport
  Theta_point 2_M : Inport  Port=2
  Theta_point 3_M : Inport  Port=3
  "                                                  " : Sum
  "                                                                                                              " : Sum
  Sortie 1 : Outport
  Sortie 2 : Outport  Port=2
  Sortie 3 : Outport  Port=3
  wires:
  "                                                  "/1 -> "                                                                                                              "/1, Sortie 2/1
  Theta_point 3_M/1 -> "                                                                                                              "/2
  Theta_point 2_M/1 -> "                                                  "/2
  Theta_point 1_M/1 -> "                                                  "/1, Sortie 1/1
  "                                                                                                              "/1 -> Sortie 3/1

== system BG/CNS/Thalamus ==
  Thetha1_estime : Inport
  Theta1_necess : Inport  Port=2
  Theta2_estime : Inport  Port=3
  Theta2_necess : Inport  Port=4
  Theta3_estime : Inport  Port=5
  Theta3_necess : Inport  Port=6
  "                              " : Sum  Inputs=-+
  "                                 " : Sum  Inputs=-+
  "                                                     " : Sum  Inputs=-+
  Saturation1 : Saturate  UpperLimit=[0 0 3*pi/4]  LowerLimit=zero_vector
  Saturation2 : Saturate  UpperLimit=[0 0 3*pi/4]  LowerLimit=zero_vector
  Saturation3 : Saturate  UpperLimit=[0 0 3*pi/4]  LowerLimit=zero_vector
  Theta_point1 : Subsystem
  theta1 : ToFile  Filename=theta1.mat  MatrixName=theta1
  theta2 : ToFile  Filename=theta2.mat  MatrixName=theta2
  theta3 : ToFile  Filename=theta3.mat  MatrixName=theta3
  Delta-theta_1 : Outport
  Delta_thetat2 : Outport  Port=2
  Delta_theta_3 : Outport  Port=3
  wires:
  "                                                     "/1 -> theta1/1, Delta-theta_1/1
  "                                 "/1 -> theta2/1, Delta_thetat2/1
  "                              "/1 -> theta3/1, Delta_theta_3/1
  Theta3_estime/1 -> "                              "/1
  Theta2_estime/1 -> "                                 "/1
  Thetha1_estime/1 -> "                                                     "/1
  Theta2_necess/1 -> "                                 "/2
  Theta1_necess/1 -> "                                                     "/2
  Theta3_necess/1 -> Theta_point1/1(In_vec), "                              "/2

== system BG/CNS/Theta1 ==
  In_vec : Inport
  Demux : Demux  Outputs=3
  x : Scope
  y : Scope
      settings: SaveName=ScopeData2
  z : Scope
      settings: SaveName=ScopeData3
  wires:
  In_vec/1 -> Demux/1
  Demux/1 -> x/1
  Demux/2 -> y/1
  Demux/3 -> z/1

== system BG/CNS/Theta2 ==
  In_vec : Inport
  Demux : Demux  Outputs=3
  x : Scope
  y : Scope
      settings: SaveName=ScopeData2
  z : Scope
      settings: SaveName=ScopeData3
  wires:
  In_vec/1 -> Demux/1
  Demux/1 -> x/1
  Demux/2 -> y/1
  Demux/3 -> z/1

== system BG/CNS/Theta3 ==
  In_vec : Inport
  Demux : Demux  Outputs=3
  x : Scope
  y : Scope
      settings: SaveName=ScopeData2
  z : Scope
      settings: SaveName=ScopeData3
  wires:
  In_vec/1 -> Demux/1
  Demux/1 -> x/1
  Demux/2 -> y/1
  Demux/3 -> z/1

== system BG/CNS/Theta_point2 ==
  In_vec : Inport
  Demux : Demux  Outputs=3
  x : Scope
  y : Scope
      settings: SaveName=ScopeData2
  z : Scope
      settings: TimeRange=2  SaveName=ScopeData3
  wires:
  In_vec/1 -> Demux/1
  Demux/1 -> x/1
  Demux/2 -> y/1
  Demux/3 -> z/1

== system BG/CNS/Vector Product  (STR1) ==
  a10 P : Inport
  a21 P : Inport  Port=2
  a32 P : Inport  Port=3
  r1 : Inport  Port=4
  r2 : Inport  Port=5
  r3 : Inport  Port=6
  Cross Product1 : vrlib/Utilities/Cross Product
  Cross Product2 : vrlib/Utilities/Cross Product
  Cross Product4 : vrlib/Utilities/Cross Product
  Integrateur : Subsystem
  Integrateur1 : Subsystem
  Integrateur2 : Subsystem
  x1 : Scope
      settings: SaveName=ScopeData7
  PV1 : Outport
  PV2 : Outport  Port=2
  PV3 : Outport  Port=3
  wires:
  Cross Product2/1 -> x1/1, PV2/1
  Cross Product1/1 -> PV1/1
  r1/1 -> Cross Product1/1
  r2/1 -> Cross Product2/1
  r3/1 -> Cross Product4/1
  Cross Product4/1 -> PV3/1
  a10 P/1 -> Integrateur/1(In1)
  a21 P/1 -> Integrateur1/1(In1)
  a32 P/1 -> Integrateur2/1(In1)
  Integrateur/1(Out1) -> Cross Product1/2
  Integrateur1/1(Out1) -> Cross Product2/2
  Integrateur2/1(Out1) -> Cross Product4/2

== system BG/CNS/st3 show ==
  In_vec : Inport
  Demux : Demux  Outputs=3
  x : Scope
  y : Scope
      settings: SaveName=ScopeData2
  z : Scope
      settings: TimeRange=2  SaveName=ScopeData3
  wires:
  In_vec/1 -> Demux/1
  Demux/1 -> x/1
  Demux/2 -> y/1
  Demux/3 -> z/1

== system BG/CNS/stn1 show ==
  In_vec : Inport
  Demux : Demux  Outputs=3
  x : Scope
  y : Scope
      settings: SaveName=ScopeData2
  z : Scope
      settings: TimeRange=2  SaveName=ScopeData3
  wires:
  In_vec/1 -> Demux/1
  Demux/1 -> x/1
  Demux/2 -> y/1
  Demux/3 -> z/1

== system BG/Monitor/OP1_ecran ==
  In_vec : Inport
  Demux : Demux  Outputs=3
  x : Scope
  y : Scope
      settings: SaveName=ScopeData2
  z : Scope
      settings: SaveName=ScopeData3
  wires:
  In_vec/1 -> Demux/1
  Demux/1 -> x/1
  Demux/2 -> y/1
  Demux/3 -> z/1

== system BG/Monitor/OP2_ecran ==
  In_vec : Inport
  Demux : Demux  Outputs=3
  x : Scope
  y : Scope
      settings: SaveName=ScopeData2
  z : Scope
      settings: SaveName=ScopeData3
  wires:
  In_vec/1 -> Demux/1
  Demux/1 -> x/1
  Demux/2 -> y/1
  Demux/3 -> z/1

== system BG/Monitor/OP3_ecran ==
  In_vec : Inport
  Demux : Demux  Outputs=3
  OP3 : simulink/Sinks/XY Graph  xmin=-0.1  xmax=1  ymin=0  ymax=1  st=-1
  x : Scope
  y : Scope
      settings: SaveName=ScopeData2
  z : Scope
      settings: SaveName=ScopeData3
  wires:
  In_vec/1 -> Demux/1
  Demux/1 -> OP3/1, x/1
  Demux/2 -> OP3/2, y/1
  Demux/3 -> z/1

== system BG/Position of segments (Forward Kinematics out of CNS)/unit_vec ==
  vec1 : Inport
  Divide : Product  Inputs=*/
  Dot Product3 : DotProduct  InputSameDT=on  OutDataTypeStr=Inherit: Inherit via internal rule
  Sqrt : Sqrt  SaturateOnIntegerOverflow=on
  vec2 : Outport
  wires:
  vec1/1 -> Divide/1, Dot Product3/2, Dot Product3/1
  Dot Product3/1 -> Sqrt/1
  Sqrt/1 -> Divide/2
  Divide/1 -> vec2/1

== system BG/Position of segments (Forward Kinematics out of CNS)/unit_vec1 ==
  vec1 : Inport
  Divide : Product  Inputs=*/
  Dot Product3 : DotProduct  InputSameDT=on  OutDataTypeStr=Inherit: Inherit via internal rule
  Sqrt : Sqrt  SaturateOnIntegerOverflow=on
  vec2 : Outport
  wires:
  vec1/1 -> Divide/1, Dot Product3/2, Dot Product3/1
  Dot Product3/1 -> Sqrt/1
  Sqrt/1 -> Divide/2
  Divide/1 -> vec2/1

== system BG/Position of segments (Forward Kinematics out of CNS)/unit_vec2 ==
  vec1 : Inport
  Divide : Product  Inputs=*/
  Dot Product3 : DotProduct  InputSameDT=on  OutDataTypeStr=Inherit: Inherit via internal rule
  Sqrt : Sqrt  SaturateOnIntegerOverflow=on
  vec2 : Outport
  wires:
  vec1/1 -> Divide/1, Dot Product3/2, Dot Product3/1
  Dot Product3/1 -> Sqrt/1
  Sqrt/1 -> Divide/2
  Divide/1 -> vec2/1

== system BG/CNS/ (GPi  SNr)/Integrateur ==
  In1 : Inport
  " " : Delay  DelayLength=1  InitialCondition=theta1_0
  "  " : Sum
  "        " : Gain  Gain=dt
  Out1 : Outport
  wires:
  "        "/1 -> "  "/1
  " "/1 -> "  "/2
  In1/1 -> "        "/1
  "  "/1 -> " "/1, Out1/1

== system BG/CNS/ (GPi  SNr)/Integrateur1 ==
  In1 : Inport
  " " : Delay  DelayLength=1  InitialCondition=theta2_0
  "  " : Sum
  "        " : Gain  Gain=dt
  Out1 : Outport
  wires:
  "        "/1 -> "  "/1
  " "/1 -> "  "/2
  In1/1 -> "        "/1
  "  "/1 -> " "/1, Out1/1

== system BG/CNS/ (GPi  SNr)/Integrateur2 ==
  In1 : Inport
  " " : Delay  DelayLength=1  InitialCondition=theta3_0
  "  " : Sum
  "        " : Gain  Gain=dt
  Out1 : Outport
  wires:
  "        "/1 -> "  "/1
  " "/1 -> "  "/2
  In1/1 -> "        "/1
  "  "/1 -> " "/1, Out1/1

== system BG/CNS/ Striosom//SNc2/Optimiseur ==
  v : Inport
  a1 : Inport  Port=2
  a2 : Inport  Port=3
  a3 : Inport  Port=4
  "                                                                                                    " : Sum  Inputs=+--
  B1 : Subsystem
  B2 : Subsystem
  Gamma1 : Subsystem
  Gamma2 : Subsystem
  lambda : Subsystem
  matrix_vector_multiplication : Subsystem
  matrix_vector_multiplication1 : Subsystem
  x : Scope
  x1 : Scope
      settings: SaveName=ScopeData4
  x2 : Scope
      settings: SaveName=ScopeData5
  v1 : Outport
  v2 : Outport  Port=2
  v3 : Outport  Port=3
  wires:
  v/1 -> "                                                                                                    "/1, matrix_vector_multiplication1/1(v1), matrix_vector_multiplication/1(v1), B2/1(v), B1/1(v), lambda/1(v)
  a1/1 -> B1/4(a1), lambda/2(a1)
  a2/1 -> B2/4(a2), lambda/3(a2)
  a3/1 -> B2/5(a3), B1/5(a3), lambda/4(a3)
  lambda/1(lambda1) -> B1/2(lambda1)
  lambda/3(lambda3) -> B1/3(lambda3), B2/3(lambda3)
  lambda/2(lamda2) -> B2/2(lambda2)
  B1/1(b11) -> Gamma2/5(b11_2), Gamma1/1(b11_1)
  B1/2(b12) -> Gamma2/6(b12_2), Gamma1/2(b12_1)
  B1/3(b21) -> Gamma2/7(b21_2), Gamma1/3(b21_1)
  B1/4(b22) -> Gamma2/8(b22_2), Gamma1/4(b22_1)
  B2/1(b11) -> Gamma1/5(b11_2), Gamma2/1(b11_1)
  B2/2(b12) -> Gamma1/6(b12_2), Gamma2/2(b12_1)
  B2/3(b21) -> Gamma1/7(b21_2), Gamma2/3(b21_1)
  B2/4(b22) -> Gamma2/4(b22_1), Gamma1/8(b22_2)
  Gamma1/1(gamma11) -> matrix_vector_multiplication/2(a11)
  Gamma1/2(gamma12) -> matrix_vector_multiplication/3(a12)
  Gamma1/3(gamma21) -> matrix_vector_multiplication/4(a21)
  Gamma1/4(gamma22) -> matrix_vector_multiplication/5(a22)
  Gamma2/1(gamma11) -> matrix_vector_multiplication1/2(a11)
  Gamma2/2(gamma12) -> matrix_vector_multiplication1/3(a12)
  Gamma2/3(gamma21) -> matrix_vector_multiplication1/4(a21)
  Gamma2/4(gamma22) -> matrix_vector_multiplication1/5(a22)
  "                                                                                                    "/1 -> v3/1
  matrix_vector_multiplication/1(vec_out) -> x/1, "                                                                                                    "/2, v1/1
  matrix_vector_multiplication1/1(vec_out) -> "                                                                                                    "/3, x1/1, v2/1
